simulink model "iterative_learning_control"  (R2024a)
settings: Solver=VariableStepAuto  StartTime=0.0  StopTime=10  RelTol=1e-3
libraries: simulink x1
settings Model: Creator=gujun  LastModifiedBy=gujun

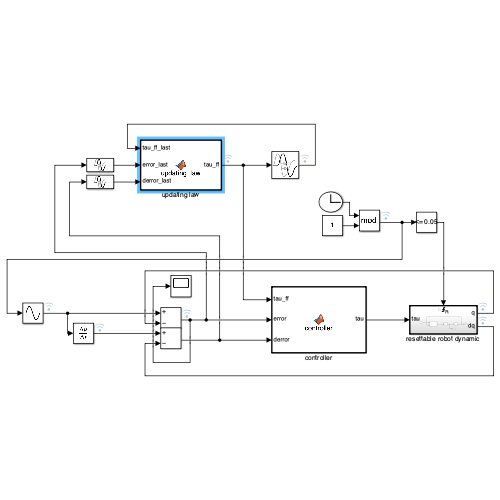
[thumbnail: Simulink's stored preview of the top-level diagram]
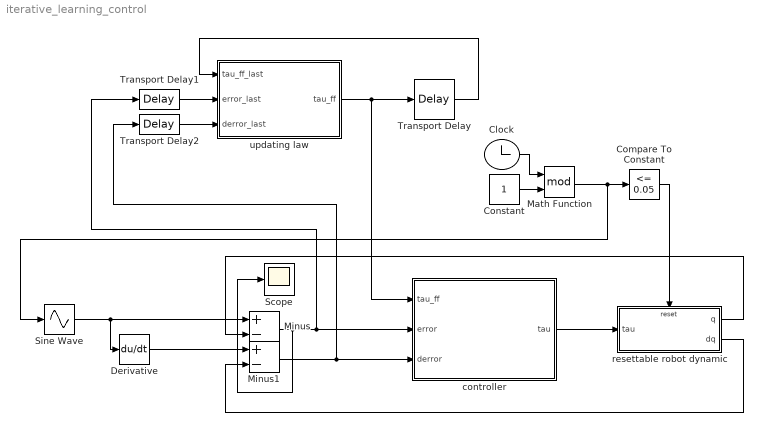
== system iterative_learning_control ==
  Clock : Clock
  Compare To Constant : simulink/Logic and Bit Operations/Compare To Constant  relop=<=  const=0.05  OutDataTypeStr=boolean
  Constant : Constant  SampleTime=-1
  Derivative : Derivative
  Math Function : Math  Operator=mod
  Minus : Sum  Inputs=+-
  Minus1 : Sum  Inputs=+-
  Scope : Scope
  Sine Wave : Sin  TimeSource=Use external signal  Frequency=2*pi  Phase=pi/2  SampleTime=0
  Transport Delay : TransportDelay
  Transport Delay1 : TransportDelay
  Transport Delay2 : TransportDelay
  controller : MATLAB Function  TreatAsAtomicUnit=on
  resettable robot dynamic : Subsystem  TreatAsAtomicUnit=on
  updating law : MATLAB Function  TreatAsAtomicUnit=on
  wires:
  Minus1/1 -> controller/3(derror), Transport Delay2/1
  updating law/1(tau_ff) -> controller/1(tau_ff), Transport Delay/1
  Transport Delay/1 -> updating law/1(tau_ff_last)
  Transport Delay1/1 -> updating law/2(error_last)
  Transport Delay2/1 -> updating law/3(derror_last)
  controller/1(tau) -> resettable robot dynamic/1(tau)
  resettable robot dynamic/2(dq) -> Minus1/2
  resettable robot dynamic/1(q) -> Minus/2
  Constant/1 -> Math Function/2
  Clock/1 -> Math Function/1
  Math Function/1 -> Sine Wave/1, Compare To Constant/1
  Compare To Constant/1 -> resettable robot dynamic/Reset
  Minus/1 -> Scope/1, Transport Delay1/1, controller/2(error)
  Sine Wave/1 -> Derivative/1, Minus/1
  Derivative/1 -> Minus1/1

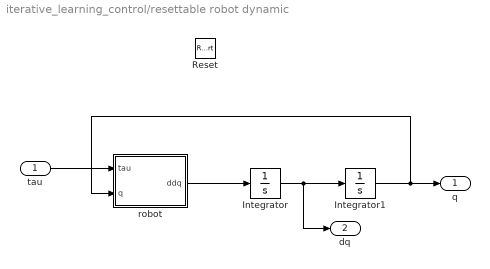
== system iterative_learning_control/resettable robot dynamic ==
  tau : Inport
  Reset : ResetPort  DisableCoverage=on
  Integrator : Integrator
  Integrator1 : Integrator
  robot : MATLAB Function  TreatAsAtomicUnit=on
  q : Outport
  dq : Outport  Port=2
  wires:
  Integrator/1 -> dq/1, Integrator1/1
  Integrator1/1 -> q/1, robot/2(q)
  robot/1(ddq) -> Integrator/1
  tau/1 -> robot/1(tau)

== matlab function iterative_learning_control/controller ==
  data: tau_ff input; error input; tau output; derror input
function tau = controller(tau_ff, error, derror)

kp = 200;


kv = 1;

tau = tau_ff + kp * error + kv * derror;

== matlab function iterative_learning_control/updating law ==
  data: tau_ff_last input; tau_ff output; error_last input; derror_last input
function tau_ff = updating_law(tau_ff_last, error_last, derror_last)

alpha = 0.5;

beta = 20;

tau_ff = tau_ff_last + alpha * (beta * error_last + derror_last);

end

== matlab function iterative_learning_control/resettable robot dynamic/robot ==
  data: tau input; ddq output; q input
function ddq = robot(tau, q)

I = 0.01;

m = 0.5;

lg = 0.2;

g = 9.8;

Ibar = I + m * lg * lg;

tauBar = tau - m * g * lg * cos(q);

ddq = tauBar / Ibar;
